simulink model "quest_initial_state"  (R2025a)
settings: Solver=ode4  StartTime=0.0  StopTime=1  FixedStep=1.0  RelTol=1e-3
model workspace (MAT data in the model file):
  step_size = 1
values from neighbouring files (symbols this model uses):
  ET0 = cspice_str2et(Date_UTC)    [initfun_18072025.m]    (also in initfun_18072025_nogyro.m)
  FOV = 166    [initfun_18072025.m]    (also in initfun_18072025_nogyro.m)
  initial_position = [-805.2933204511233 , -515.0283481792998, 6924.330181946009 ]    [initfun_18072025.m]    (also in initfun_18072025_nogyro.m)
  K = [F Z(:); Z(:)' sigma]    [Gain_matrix.m]    (also in QUEST.m = Gain_matrix(V',W',a); initfun_18072025.m = schmidt(nmax, mmax); initfun_18072025_nogyro.m = schmidt(nmax, mmax))
  Magnetometers_number = 2    [initfun_18072025.m]    (also in initfun_18072025_nogyro.m)
  Mean_cart_Mag = 0    [initfun_18072025.m]    (also in initfun_18072025_nogyro.m)
  MeanangularSun = 0    [initfun_18072025.m]    (also in initfun_18072025_nogyro.m)
  mmax = 3    [initfun_18072025.m]    (also in initfun_18072025_nogyro.m)
  nmax = 3    [initfun_18072025.m]    (also in initfun_18072025_nogyro.m)
  Sigma_cart_Mag = (50*10^-9)/3    (= 1.66666666667e-08)    [initfun_18072025.m]    (also in initfun_18072025_nogyro.m)
  SigmaangularSun = 0.1    [initfun_18072025.m]    (also in initfun_18072025_nogyro.m)
  Sun_sensors = zeros(3, SS_number)    [initfun_18072025.m]    (also in initfun_18072025_nogyro.m)
undefined symbols (not defined in the file or in its folder): G, H, IAU, juliandate, quat_0
libraries: aerolibtransform2 x1
settings Model: Creator=pietr  LastModifiedBy=pietr

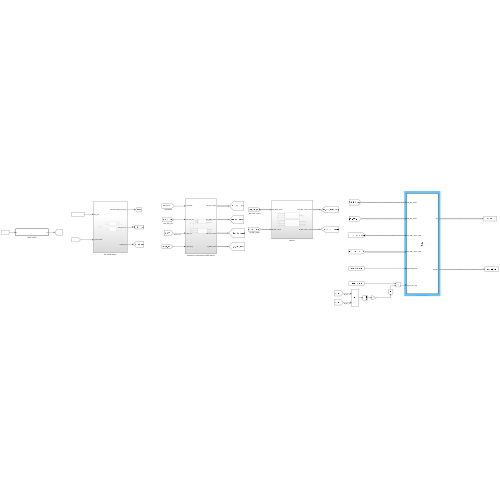
[thumbnail: Simulink's stored preview of the top-level diagram]
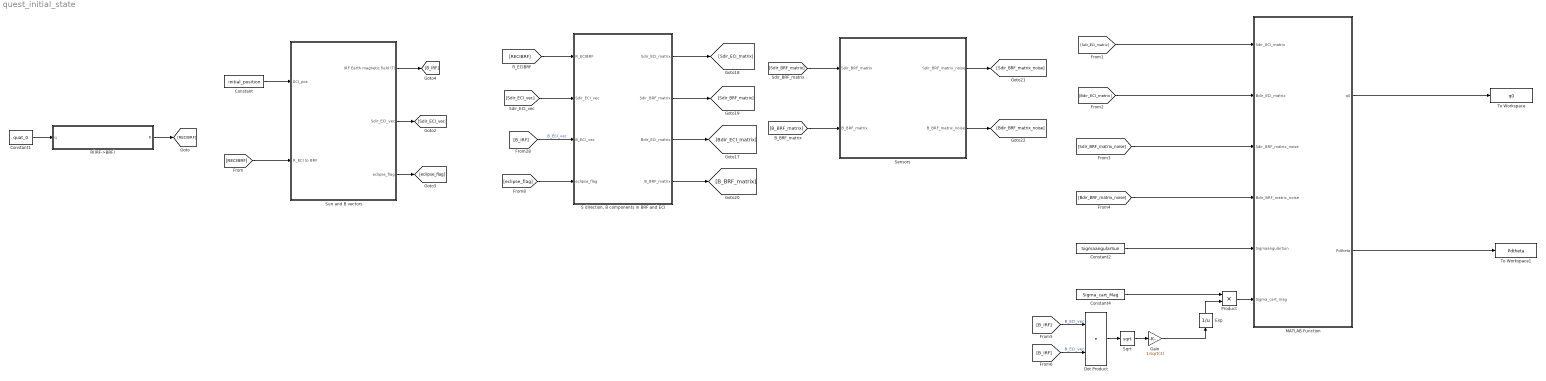
== system quest_initial_state ==
  Constant : Constant  Value=initial_position
  Constant1 : Constant  Value=quat_0
  Constant2 : Constant  Value=SigmaangularSun
  Constant4 : Constant  Value=Sigma_cart_Mag
  Dot Product : DotProduct  OutDataTypeStr=Inherit: Inherit via internal rule
  Exp : Math  Operator=reciprocal
  Gain : Gain  Gain=1/sqrt(3)
  MATLAB Function : MATLAB Function  TreatAsAtomicUnit=on  SystemSampleTime=step_size
  Product : Product
  R(IRF->BRF) : MATLAB Function  TreatAsAtomicUnit=on
  "S direction, B components in BRF and ECI" : Subsystem
  Sensors : Subsystem
  Sqrt : Sqrt
  Sun and B vectors : Subsystem
  To Workspace : ToWorkspace  VariableName=q0  SaveFormat=Structure  SampleTime=-1
  To Workspace1 : ToWorkspace  VariableName=Pdtheta  SaveFormat=Structure  SampleTime=-1
  wires:
  [B_BRF_matrix] -> Sensors/2(B_BRF_matrix)
  "S direction, B components in BRF and ECI"/4(B_BRF_matrix) -> [B_BRF_matrix]
  [RECIBRF] -> "S direction, B components in BRF and ECI"/1(R_ECIBRF)
  [B_IRF] -> "S direction, B components in BRF and ECI"/3(B_ECI_vec)  "B_ECI_vec"
  [Sdir_ECI_vec] -> "S direction, B components in BRF and ECI"/2(Sdir_ECI_vec)
  "S direction, B components in BRF and ECI"/3(Bdir_ECI_matrix) -> [Bdir_ECI_matrix]
  "S direction, B components in BRF and ECI"/1(Sdir_ECI_matrix) -> [Sdir_ECI_matrix]
  [Sdir_BRF_matrix] -> Sensors/1(Sdir_BRF_matrix)
  "S direction, B components in BRF and ECI"/2(Sdir_BRF_matrix) -> [Sdir_BRF_matrix]
  [eclipse_flag] -> "S direction, B components in BRF and ECI"/4(eclipse_flag)
  Sensors/2(B_BRF_matrix_noise) -> [Bdir_BRF_matrix_noise]
  Sensors/1(Sdir_BRF_matrix_noise) -> [Sdir_BRF_matrix_noise]
  Constant1/1 -> R(IRF->BRF)/1(q)
  R(IRF->BRF)/1(R) -> [RECIBRF]
  Constant/1 -> Sun and B vectors/1(ECI_pos)
  [RECIBRF] -> Sun and B vectors/2(R_ECI to BRF)
  Sun and B vectors/3(eclipse_flag) -> [eclipse_flag]
  Sun and B vectors/2(Sdir_ECI_vec) -> [Sdir_ECI_vec]
  Sun and B vectors/1(IRF Earth magnetic field (T)) -> [B_IRF]
  [Sdir_ECI_matrix] -> MATLAB Function/1(Sdir_ECI_matrix)
  [Bdir_ECI_matrix] -> MATLAB Function/2(Bdir_ECI_matrix)
  [Sdir_BRF_matrix_noise] -> MATLAB Function/3(Sdir_BRF_matrix_noise)
  [Bdir_BRF_matrix_noise] -> MATLAB Function/4(Bdir_BRF_matrix_noise)
  Constant4/1 -> Product/1
  Constant2/1 -> MATLAB Function/5(SigmaangularSun)
  [B_IRF] -> Dot Product/1  "B_ECI_vec"
  [B_IRF] -> Dot Product/2  "B_ECI_vec"
  Dot Product/1 -> Sqrt/1
  Sqrt/1 -> Gain/1
  Gain/1 -> Exp/1
  Exp/1 -> Product/2
  Product/1 -> MATLAB Function/6(Sigma_cart_mag)
  MATLAB Function/1(q0) -> To Workspace/1
  MATLAB Function/2(Pdtheta) -> To Workspace1/1

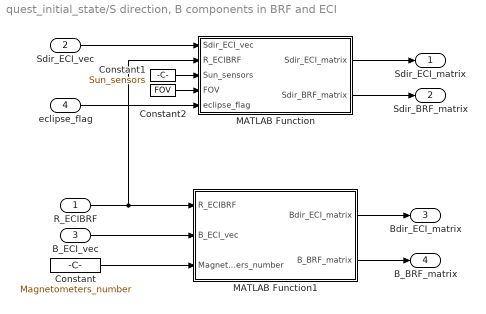
== system quest_initial_state/S direction, B components in BRF and ECI ==
  R_ECIBRF : Inport
  Sdir_ECI_vec : Inport  Port=2
  B_ECI_vec : Inport  Port=3
  eclipse_flag : Inport  Port=4
  Constant : Constant  Value=Magnetometers_number
  Constant1 : Constant  Value=Sun_sensors
  Constant2 : Constant  Value=FOV
  MATLAB Function : MATLAB Function  TreatAsAtomicUnit=on  SystemSampleTime=step_size
  MATLAB Function1 : MATLAB Function  TreatAsAtomicUnit=on  SystemSampleTime=step_size
  Sdir_ECI_matrix : Outport
  Sdir_BRF_matrix : Outport  Port=2
  Bdir_ECI_matrix : Outport  Port=3
  B_BRF_matrix : Outport  Port=4
  wires:
  Sdir_ECI_vec/1 -> MATLAB Function/1(Sdir_ECI_vec)
  R_ECIBRF/1 -> MATLAB Function1/1(R_ECIBRF), MATLAB Function/2(R_ECIBRF)
  B_ECI_vec/1 -> MATLAB Function1/2(B_ECI_vec)
  MATLAB Function/1(Sdir_ECI_matrix) -> Sdir_ECI_matrix/1
  MATLAB Function/2(Sdir_BRF_matrix) -> Sdir_BRF_matrix/1
  MATLAB Function1/1(Bdir_ECI_matrix) -> Bdir_ECI_matrix/1
  MATLAB Function1/2(B_BRF_matrix) -> B_BRF_matrix/1
  Constant/1 -> MATLAB Function1/3(Magnetometers_number)
  Constant1/1 -> MATLAB Function/3(Sun_sensors)
  Constant2/1 -> MATLAB Function/4(FOV)
  eclipse_flag/1 -> MATLAB Function/5(eclipse_flag)

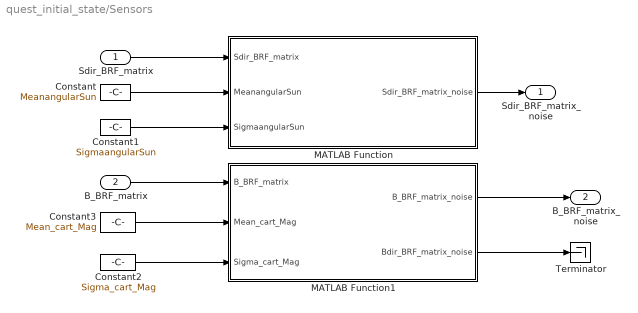
== system quest_initial_state/Sensors ==
  Sdir_BRF_matrix : Inport
  B_BRF_matrix : Inport  Port=2
  Constant : Constant  Value=MeanangularSun
  Constant1 : Constant  Value=SigmaangularSun
  Constant2 : Constant  Value=Sigma_cart_Mag
  Constant3 : Constant  Value=Mean_cart_Mag
  MATLAB Function : MATLAB Function  TreatAsAtomicUnit=on  SystemSampleTime=step_size
  MATLAB Function1 : MATLAB Function  TreatAsAtomicUnit=on  SystemSampleTime=step_size
  Terminator : Terminator
  Sdir_BRF_matrix_noise : Outport
  B_BRF_matrix_noise : Outport  Port=2
  wires:
  Sdir_BRF_matrix/1 -> MATLAB Function/1(Sdir_BRF_matrix)
  B_BRF_matrix/1 -> MATLAB Function1/1(B_BRF_matrix)
  MATLAB Function/1(Sdir_BRF_matrix_noise) -> Sdir_BRF_matrix_noise/1
  Constant/1 -> MATLAB Function/2(MeanangularSun)
  Constant1/1 -> MATLAB Function/3(SigmaangularSun)
  Constant2/1 -> MATLAB Function1/3(Sigma_cart_Mag)
  Constant3/1 -> MATLAB Function1/2(Mean_cart_Mag)
  MATLAB Function1/1(B_BRF_matrix_noise) -> B_BRF_matrix_noise/1
  MATLAB Function1/2(Bdir_BRF_matrix_noise) -> Terminator/1

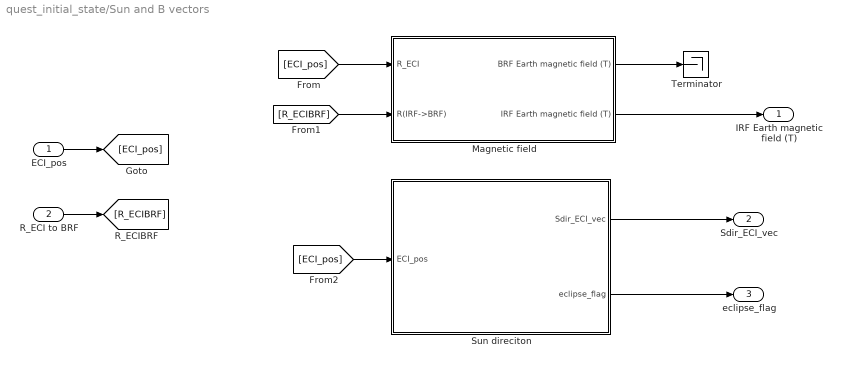
== system quest_initial_state/Sun and B vectors ==
  ECI_pos : Inport
  R_ECI to BRF : Inport  Port=2
  Magnetic field : Subsystem
  Sun direciton : Subsystem
  Terminator : Terminator
  IRF Earth magnetic field (T) : Outport
  Sdir_ECI_vec : Outport  Port=2
  eclipse_flag : Outport  Port=3
  wires:
  Magnetic field/2(IRF Earth magnetic field (T)) -> IRF Earth magnetic field (T)/1
  ECI_pos/1 -> [ECI_pos]
  R_ECI to BRF/1 -> [R_ECIBRF]
  [ECI_pos] -> Magnetic field/1(R_ECI)
  [R_ECIBRF] -> Magnetic field/2(R(IRF->BRF))
  [ECI_pos] -> Sun direciton/1(ECI_pos)
  Sun direciton/1(Sdir_ECI_vec) -> Sdir_ECI_vec/1
  Sun direciton/2(eclipse_flag) -> eclipse_flag/1
  Magnetic field/1("BRF Earth magnetic field (T)  ") -> Terminator/1

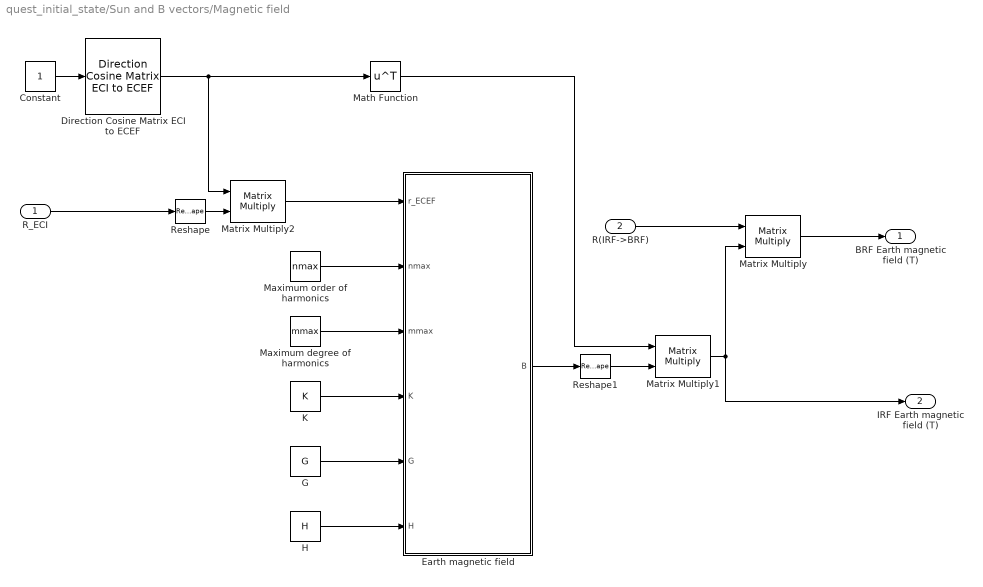
== system quest_initial_state/Sun and B vectors/Magnetic field ==
  R_ECI : Inport
  R(IRF->BRF) : Inport  Port=2
  Constant : Constant
  Direction Cosine Matrix ECI to ECEF : aerolibtransform2/Direction Cosine Matrix ECI to ECEF  red=IAU-2000/2006  year=2025  month=July  day=23  hour=8  min=30  sec=0  deltaT=Sec  errorflag=Error  extraparamflag=off
      settings: AttributesFormatString=%<red>
  "Earth magnetic field " : MATLAB Function  TreatAsAtomicUnit=on
  G : Constant  Value=G  VectorParams1D=off
  H : Constant  Value=H  VectorParams1D=off
  K : Constant  Value=K  VectorParams1D=off
  Math Function : Math  Operator=transpose  SignedPower=on
  Matrix Multiply : Product  Multiplication=Matrix(*)
  Matrix Multiply1 : Product  Multiplication=Matrix(*)
  Matrix Multiply2 : Product  Multiplication=Matrix(*)
  "Maximum degree of harmonics " : Constant  Value=mmax
  "Maximum order of harmonics " : Constant  Value=nmax
  Reshape : Reshape  OutputDimensionality=Column vector (2-D)
  Reshape1 : Reshape  OutputDimensionality=Column vector (2-D)
  "BRF Earth magnetic field (T)  " : Outport
  IRF Earth magnetic field (T) : Outport  Port=2
  wires:
  R_ECI/1 -> Reshape/1
  H/1 -> "Earth magnetic field "/6(H)
  Reshape/1 -> Matrix Multiply2/2
  "Maximum order of harmonics "/1 -> "Earth magnetic field "/2(nmax)
  R(IRF->BRF)/1 -> Matrix Multiply/1
  Matrix Multiply1/1 -> IRF Earth magnetic field (T)/1, Matrix Multiply/2
  Matrix Multiply2/1 -> "Earth magnetic field "/1(r_ECEF)
  "Earth magnetic field "/1(B) -> Reshape1/1
  "Maximum degree of harmonics "/1 -> "Earth magnetic field "/3(mmax)
  Math Function/1 -> Matrix Multiply1/1
  Reshape1/1 -> Matrix Multiply1/2
  Constant/1 -> Direction Cosine Matrix ECI to ECEF/1
  K/1 -> "Earth magnetic field "/4(K)
  Matrix Multiply/1 -> "BRF Earth magnetic field (T)  "/1
  G/1 -> "Earth magnetic field "/5(G)
  Direction Cosine Matrix ECI to ECEF/1 -> Matrix Multiply2/1, Math Function/1

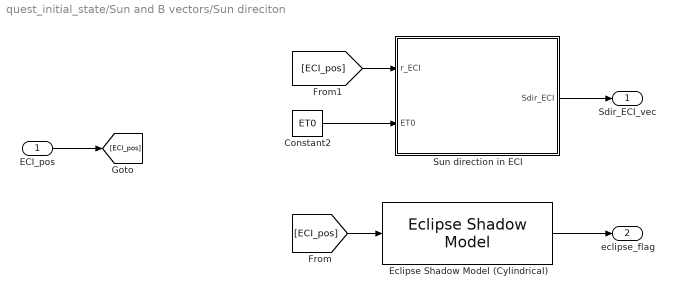
== system quest_initial_state/Sun and B vectors/Sun direciton ==
  ECI_pos : Inport
  Constant2 : Constant  Value=ET0
  Eclipse Shadow Model (Cylindrical) : EclipseShadowModel  units=Metric (km)  shadowModel=Cylindrical  startDate=juliandate(2025, 7, 23, 8, 30, 00)  includeMoon=off  ephemerisModel=DE430  useEphemerisDateRange=off
  Sun direction in ECI : MATLAB Function  TreatAsAtomicUnit=on
  Sdir_ECI_vec : Outport
  eclipse_flag : Outport  Port=2
  wires:
  Constant2/1 -> Sun direction in ECI/2(ET0)
  ECI_pos/1 -> [ECI_pos]
  [ECI_pos] -> Eclipse Shadow Model (Cylindrical)/1
  [ECI_pos] -> Sun direction in ECI/1(r_ECI)
  Eclipse Shadow Model (Cylindrical)/1 -> eclipse_flag/1
  Sun direction in ECI/1(Sdir_ECI) -> Sdir_ECI_vec/1

== matlab function quest_initial_state/MATLAB Function ==
  data: Sdir_ECI_matrix input; Bdir_ECI_matrix input; Sdir_BRF_matrix_noise input; Bdir_BRF_matrix_noise input; SigmaangularSun input; q0 output; Sigma_cart_mag input; Pdtheta output
function [q0,Pdtheta] = fcn(Sdir_ECI_matrix, Bdir_ECI_matrix, Sdir_BRF_matrix_noise, Bdir_BRF_matrix_noise, SigmaangularSun, Sigma_cart_mag)
%% QUEST
q0 = zeros(4,1);
SS = size(Sdir_ECI_matrix,2);
MM = size(Bdir_ECI_matrix,2);

ECI_directions = [Sdir_ECI_matrix, Bdir_ECI_matrix];
BRF_directions = [Sdir_BRF_matrix_noise, Bdir_BRF_matrix_noise];

% angle = acosd(dot(Sdir_ECI_matrix(:,1),Bdir_ECI_matrix(:,1)));
% disp(angle);
n_vec = size(ECI_directions,2);
q0 = QUEST(ECI_directions',BRF_directions',ones(1,n_vec));

SigmaangularSun = deg2rad(SigmaangularSun);

sigmatot = 1/ sqrt(SS/(SigmaangularSun)^2 + MM/(sqrt(3)*Sigma_cart_mag)^2); % Come Sigma_cart_mag si è scelto il valore da datasheet lungo i 3 assi, ma normalizzato.
a = zeros(SS+MM,1);
a(1:SS) = sigmatot^2 / SigmaangularSun^2; 
a(SS+1:end) = sigmatot^2 / (sqrt(3)*Sigma_cart_mag)^2;

sum=zeros(3,3);
for i=1:n_vec
    sum = sum + a(i)*BRF_directions(:,i)*BRF_directions(:,i)';
end
Pdtheta = zeros(3,3);
Pdtheta=sigmatot^2.*((eye(3)-sum)^-1);

end

== matlab function quest_initial_state/Sun and B vectors/Magnetic field/Earth magnetic field  ==
  data: r_ECEF input; B output; nmax input; mmax input; K input; G input; H input
function B = fcn(r_ECEF, nmax, mmax, K, G, H)

R_mean = 6371.2; % Mean radius for International Geomagnetic Reference Field
e1 = [1 0 0];
e2 = [0 1 0];
e3 = [0 0 1];

A = zeros(nmax+3, mmax+3);
ctilde = zeros(nmax+3,1);
stilde = zeros(nmax+3,1);

[A, ctilde, stilde] = recursion(r_ECEF, nmax, mmax);

rho = norm(r_ECEF);
r_vers = r_ECEF'/rho;

u = r_vers(3); % argumento of latitude
B = [0 0 0];

scalar = (R_mean/rho)^2;
ttilde = G;
b1 = ttilde;
b2 = ttilde;
b3 = ttilde;
br = ttilde;
for n=1:nmax
    
   scalar = scalar*R_mean/rho;
   
   i = n+1;
    for m =0:n 
        
        j = m+1;
        
        if m <= mmax
            ttilde(i,j) = G(i,j)*ctilde(j) + H(i,j)*stilde(j);
            
            b3(i,j) =  -ttilde(i,j)*A(i,j+1);
            
            br(i,j) = ttilde(i,j)*(u*A(i,j+1) + (n+m+1)*A(i,j));
            
            B = B + scalar*K(i,j)*(b3(i,j)*e3 + br(i,j)*r_vers);
        end 
        
    if ((m > 0) && (m <= mmax))
        
        b1(i,j) = -m*A(i,j)*(G(i,j)*ctilde(j-1) + H(i,j)*stilde(j-1));
        
        b2(i,j) = -m*A(i,j)*(H(i,j)*ctilde(j-1) - G(i,j)*stilde(j-1));
        
        B = B + scalar*K(i,j)*(b1(i,j)*e1 + b2(i,j)*e2);
    end 
    end 

end
end

function [A, ctilde, stilde] = recursion(r, nmax, mmax)
A = zeros(nmax+3, mmax+3);

R_m = norm(r);
rhat = r./R_m;
u = rhat(3);

A(1,1) = 1;
A(2,1) = u;
A(2,2) = 1;

ctilde = zeros(nmax+3,1);
stilde = zeros(nmax+3,1);

ctilde(1) = 1;
ctilde(2) = rhat(1);
stilde(1) = 0;
stilde(2) = rhat(2);

for n = 2:nmax
    i = n+1;
    
    A(i,i) = prod(1:2:(2*n-1));
    A(i,i-1) = u*A(i,i);
    
    if n<=nmax
        
        ctilde(i) = ctilde(2) * ctilde(i-1) - stilde(2) * stilde(i-1);
        stilde(i)  = stilde(2) * ctilde(i-1) + ctilde(2) * stilde(i-1);
        
    end
  for m = 0:n
      
    j=m+1;
    
    if (m < (n-1)) && (m <= (mmax+1))
        
      A(i,j)=((2*n - 1)*u*A((i-1),j) - (n+m-1)*A((i-2),j))/(n-m);
      
    end

  end
end 
end

== matlab function quest_initial_state/Sun and B vectors/Sun direciton/Sun direction in ECI ==
  data: r_ECI input; Sdir_ECI output; ET0 input
function Sdir_ECI = fcn(r_ECI, ET0)

ET = ET0;
coder.extrinsic('cspice_spkpos');
% Preallocazione necessaria perché Simulink non sa che output aspettarsi
R_ESun_ECI = zeros(3,1);

[R_ESun_ECI, ~] = cspice_spkpos('SUN', ET, 'J2000', 'NONE', 'EARTH'); % Sun position in ECI wrt earth

R_SatSun_ECI = R_ESun_ECI - r_ECI(:); % Sun position wrt the sat in ECI
Sdir_ECI = R_SatSun_ECI/norm(R_SatSun_ECI); % Sun direction wrt sat ECI
end

== matlab function quest_initial_state/R(IRF->BRF) ==
  data: q input; R output
function R = R_by_q(q)

%% Description 
% This block provides the rotation matrix corresponding to the quaternion
% in input. THE SCALAR LAST CONVENTION IS USED FOR THE QUATERNION

%% INPUT 
% q -> 4x1 array (quaternion)
%% OUTPUT 
% R -> 3x3 matrix (rotation matrix)
q = q / norm(q); 
q0 = q(4); 
q1 = q(1);
q2 = q(2);
q3 = q(3);

R = [q0^2+q1^2-q2^2-q3^2 2*q1*q2+2*q0*q3 2*q1*q3-2*q0*q2;
    2*q1*q2-2*q0*q3 q0^2-q1^2+q2^2-q3^2 2*q2*q3+2*q0*q1;
    2*q1*q3+2*q0*q2 2*q2*q3-2*q0*q1 q0^2-q1^2-q2^2+q3^2];
end

== matlab function quest_initial_state/Sensors/MATLAB Function ==
  data: Sdir_BRF_matrix input; Sdir_BRF_matrix_noise output; MeanangularSun input; SigmaangularSun input
function Sdir_BRF_matrix_noise = noiseSun(Sdir_BRF_matrix, MeanangularSun, ...
    SigmaangularSun)


sizeS = size(Sdir_BRF_matrix);
s = sizeS(2);

if s == 0
    Sdir_BRF_matrix_noise = [];
else
    Sdir_BRF_matrix_noise = zeros(sizeS);
    
    s_true = Sdir_BRF_matrix(:,1);
    s_true = s_true(:);
    
    for i = 1:s   
        Alpha_s=deg2rad(MeanangularSun)+randn(1).*deg2rad(SigmaangularSun); %radians
        Beta_s=rand(1).*2*pi; %radians
    
        if s_true==[1;0;0]    
            k_s=[0 0 1]';
        else
            k_s=[1 0 0]';
        end
        
        h_s=cross(s_true,k_s)./norm(cross(s_true,k_s));
        g_s=s_true.*cos(Alpha_s)+cross(h_s,s_true).*sin(Alpha_s);
        s_mes=g_s.*cos(Beta_s)+cross(s_true,g_s).*sin(Beta_s)+s_true.*dot(s_true,g_s).*(1-cos(Beta_s));
    
        if norm(s_mes)-1 >10e-10    
            disp('warning')
            s_mes = s_mes/norm(s_mes);
        end
    
        Sdir_BRF_matrix_noise(:,i) = s_mes/norm(s_mes); 
    end
end

== matlab function quest_initial_state/Sensors/MATLAB Function1 ==
  data: B_BRF_matrix input; Mean_cart_Mag input; Sigma_cart_Mag input; B_BRF_matrix_noise output; Bdir_BRF_matrix_noise output
function [B_BRF_matrix_noise, Bdir_BRF_matrix_noise] = noiseMag(B_BRF_matrix, Mean_cart_Mag, ...
    Sigma_cart_Mag)

sizeB = size(B_BRF_matrix);
t = sizeB(2);
Bdir_BRF_matrix_noise = zeros(sizeB);
B_BRF_matrix_noise = zeros (sizeB);

B_true = B_BRF_matrix(:,1);
B_true = B_true(:);
B_meas = zeros(3,1);

for j = 1:t 
    B_meas = B_BRF_matrix(:,j) + randn(3,1)*Sigma_cart_Mag;
    B_BRF_matrix_noise(:,j) = B_meas;
    Bdir_BRF_matrix_noise(:,j) = B_meas / norm(B_meas);
end
end

== matlab function quest_initial_state/S direction, B components in BRF and ECI/MATLAB Function ==
  data: Sdir_ECI_vec input; R_ECIBRF input; Sdir_ECI_matrix output; Sdir_BRF_matrix output; Sun_sensors input; FOV input; eclipse_flag input
function [Sdir_ECI_matrix, Sdir_BRF_matrix] = fcn(Sdir_ECI_vec, R_ECIBRF, ...
    Sun_sensors, FOV, eclipse_flag)

if eclipse_flag == 0
    Sdir_ECI_matrix = [];
    Sdir_BRF_matrix = [];
else    
    Sdir_BRF_vec = R_ECIBRF*Sdir_ECI_vec; % Sun direction wrt satellite in the BRF
    
    temp_ECI = zeros(3,length(Sun_sensors(1,:)));
    temp_BRF = zeros(3,length(Sun_sensors(1,:)));
    visible = false(1, length(Sun_sensors(1,:))); 
    
    % Visibility check in sunlight
    for i = 1 : length(Sun_sensors(1,:))
    
        cos_theta = dot(Sdir_BRF_vec, Sun_sensors(:,i)); % where theta is the angle between the normal to the i-th Sun sensor and the Sun direction, both in the BRF
        
        if cos_theta > cosd(FOV/2)
                
                temp_BRF(:,i) = Sdir_BRF_vec/norm(Sdir_BRF_vec);
                temp_ECI(:,i) = Sdir_ECI_vec/norm(Sdir_ECI_vec);
                visible(i) = true;
        end
    end
    
    Sdir_ECI_matrix = temp_ECI(:, visible);
    Sdir_BRF_matrix = temp_BRF(:, visible);
end

end

== matlab function quest_initial_state/S direction, B components in BRF and ECI/MATLAB Function1 ==
  data: R_ECIBRF input; Bdir_ECI_matrix output; B_ECI_vec input; B_BRF_matrix output; Magnetometers_number input
function [Bdir_ECI_matrix, B_BRF_matrix] = fcn(R_ECIBRF, B_ECI_vec,...
    Magnetometers_number)

B_BRF_vec = R_ECIBRF * B_ECI_vec;

Bdir_ECI_matrix = zeros(3, Magnetometers_number);
B_BRF_matrix = zeros(3, Magnetometers_number);

for k = 1:Magnetometers_number
    Bdir_ECI_matrix(:,k) = B_ECI_vec/norm(B_ECI_vec);
    B_BRF_matrix(:,k) = B_BRF_vec;
end

end
